simulink model "risc_biloc"  (Simulink 10.0)
settings: Solver=ode15s  StartTime=0.0  StopTime=24  FixedStep=.5  RelTol=1e-4  EnableMultiTasking=on
values from neighbouring files (symbols this model uses):
  A = [-(G1+G12)/C1  G12/C1; G12/C2  -(G2+G12)/C2]    [risc_biloc_dim.m]
  B = [1/C1 0;0 1/C2]    [risc_biloc_dim.m]
  C = eye(2)    [risc_biloc_dim.m]
  D = zeros(2,3)    [risc_biloc_dim.m]
libraries: simulink x2
settings Model: Creator=prof. G. Celentano  LastModifiedBy=giuseppericcio  ExtModeTrigMode=oneshot  ExtModeArmWhenConnect=off
settings DataIOCC: SignalLoggingSaveFormat=ModelDataLogs  SignalLoggingName=sigsOut
settings OptimizationCC: BooleanDataType=off  ExpressionDepthLimit=2147483647  InitFltsAndDblsToZero=on
settings DebuggingCC: SaveWithParameterizedLinksMsg=none  SignalResolutionControl=TryResolveAllWithWarning  MultiTaskDSMMsg=warning  MultiTaskCondExecSysMsg=none  FcnCallInpInsideContextMsg=warning  StateNameClashWarn=warning
settings HardwareCC: TargetUnknown=on
settings GRTTargetCC: TargetFcnLib=ansi_tfl_tmw.mat

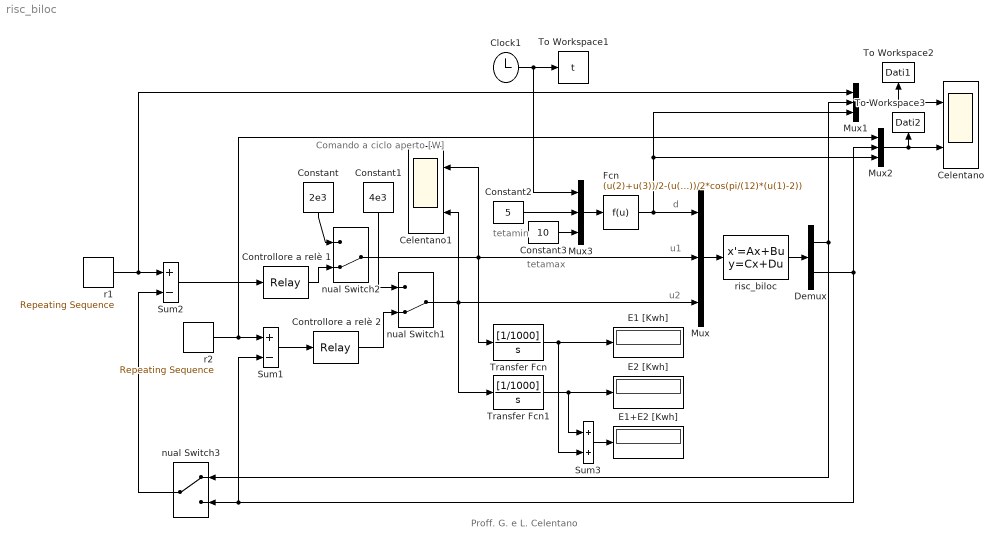
== system risc_biloc ==
  note: Comando  a
      |  ciclo aperto [W]
  note: d
  note: u2
  note: Proff. G. e L. Celentano
  note: u1
  note: tetamin
  note: tetamax
  Celentano : Scope  NumInputPorts=2
  Celentano1 : Scope  NumInputPorts=2
  Clock1 : Clock
  Constant : Constant  Value=2e3
  Constant1 : Constant  Value=4e3
  Constant2 : Constant  Value=5
  Constant3 : Constant  Value=10
  Controllore a relè 1 : Relay  OnSwitchValue=1  OffSwitchValue=-1  OnOutputValue=2000
  Controllore a relè 2 : Relay  OnSwitchValue=1  OffSwitchValue=-1  OnOutputValue=4000
  Demux : Demux  Outputs=2
  E1 [Kwh] : Display
  E1+E2 [Kwh] : Display
  E2 [Kwh] : Display
  Fcn : Fcn  Expr=(u(2)+u(3))/2-(u(3)-u(2))/2*cos(pi/(12)*(u(1)-2))
  Mux{,1..3} (4 alike) : Mux  Inputs=3
  Sum1 : Sum  Inputs=+-  SaturateOnIntegerOverflow=on  InputSameDT=on  OutDataTypeStr=Inherit: Same as first input
  Sum2 : Sum  Inputs=+-  SaturateOnIntegerOverflow=on  InputSameDT=on  OutDataTypeStr=Inherit: Same as first input
  Sum3 : Sum  SaturateOnIntegerOverflow=on  InputSameDT=on  OutDataTypeStr=Inherit: Same as first input
  To Workspace1 : ToWorkspace  VariableName=t  SampleTime=-1
  To Workspace2 : ToWorkspace  VariableName=Dati1  SampleTime=-1
  To Workspace3 : ToWorkspace  VariableName=Dati2  SampleTime=-1
  Transfer Fcn : TransferFcn  Numerator=[1/1000]  Denominator=[1 0]
  Transfer Fcn1 : TransferFcn  Numerator=[1/1000]  Denominator=[1 0]
  nual Switch1 : ManualSwitch  CurrentSetting=0
  nual Switch2 : ManualSwitch  CurrentSetting=0
  nual Switch3 : ManualSwitch
  r1 : simulink/Sources/Repeating Sequence  rep_seq_t=[0 7 7.5 9.5 10 17 17.5 21.5 22 24]  rep_seq_y=[0 0 4 4 0 0 4 4 0 0]+16
  r2 : simulink/Sources/Repeating Sequence  rep_seq_t=[0 7 7.5 9.5 10 17 17.5 21.5 22 24]  rep_seq_y=[0 0 4 4 0 0 4 4 0 0]+18
  risc_biloc : StateSpace  A=A*60*60  B=[E B]*60*60  C=C  D=D  InitialCondition=[10 10]
  wires:
  Mux/1 -> risc_biloc/1
  risc_biloc/1 -> Demux/1
  nual Switch2/1 -> Transfer Fcn/1, Celentano1/1, Mux/2
  r1/1 -> Sum2/1, Mux1/1
  Mux1/1 -> To Workspace2/1, Celentano/1
  nual Switch1/1 -> Mux/3, Transfer Fcn1/1, Celentano1/2
  Controllore a relè 2/1 -> nual Switch1/2
  Controllore a relè 1/1 -> nual Switch2/2
  r2/1 -> Sum1/1, Mux2/1
  Sum1/1 -> Controllore a relè 2/1
  Constant/1 -> nual Switch2/1
  Constant1/1 -> nual Switch1/1
  Sum2/1 -> Controllore a relè 1/1
  Mux2/1 -> To Workspace3/1, Celentano/2
  Demux/1 -> Mux1/2, nual Switch3/1
  Demux/2 -> Mux2/2, Sum1/2, nual Switch3/2
  Transfer Fcn/1 -> E1 [Kwh]/1, Sum3/2
  Transfer Fcn1/1 -> E2 [Kwh]/1, Sum3/1
  Fcn/1 -> Mux2/3, Mux1/3, Mux/1
  Sum3/1 -> E1+E2 [Kwh]/1
  Constant2/1 -> Mux3/2
  Constant3/1 -> Mux3/3
  Mux3/1 -> Fcn/1
  Clock1/1 -> To Workspace1/1, Mux3/1
  nual Switch3/1 -> Sum2/2
